simulink subsystem "EncodersvAJ"  (R2023b)
settings: Solver=VariableStepAuto  StartTime=0.0  StopTime=10.0  RelTol=1e-3
libraries: arduinosensorlib x2
settings Model: Creator=USUARIO  LastModifiedBy=USUARIO

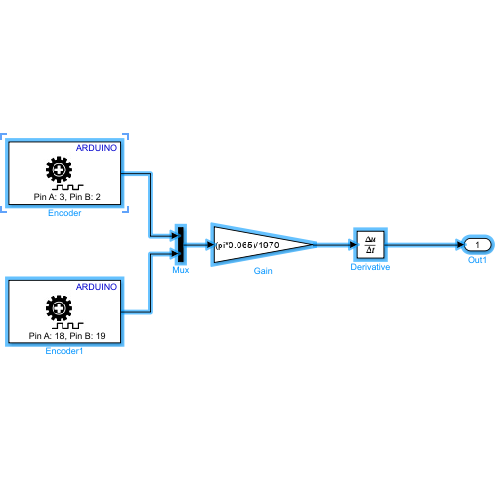
[thumbnail: Simulink's stored preview of the top-level diagram]
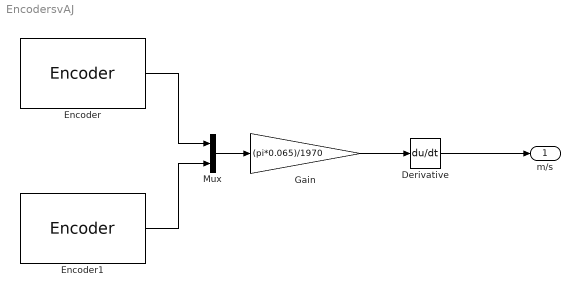
== system EncodersvAJ ==
  Derivative : Derivative
  Encoder : arduinosensorlib/Encoder  InputA=3  InputB=2  Mode=No reset  SampleTime=0.01
  Encoder1 : arduinosensorlib/Encoder  InputA=18  InputB=19  Mode=No reset  SampleTime=0.01
  Gain : Gain  Gain=(pi*0.065)/1970  OutDataTypeStr=double
  Mux : Mux  Inputs=2
  m/s : Outport
  wires:
  Gain/1 -> Derivative/1
  Mux/1 -> Gain/1
  Derivative/1 -> m/s/1
  Encoder1/1 -> Mux/2
  Encoder/1 -> Mux/1
